simulink model "mit_ctl_Harness1"  (R2023a)
settings: configuration reference "config" (kept outside this file)
settings Model: DataDictionary=model_config.sldd  Creator=Administrator  LastModifiedBy=Administrator
settings ConfigSetRef: SourceName=config

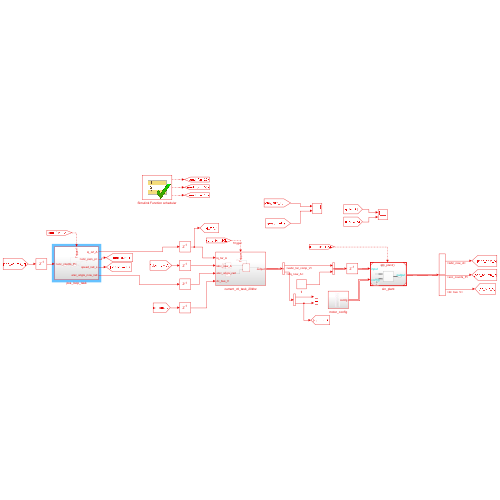
[thumbnail: Simulink's stored preview of the top-level diagram]
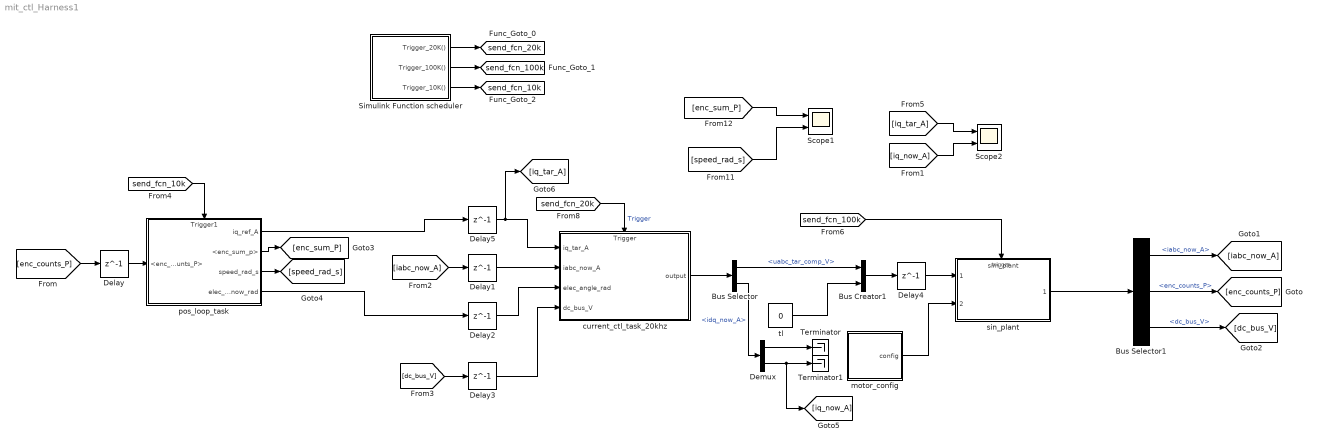
== system mit_ctl_Harness1 ==
  Bus Creator1 : BusCreator  Inputs=2  OutDataTypeStr=Bus: SimPlantInput  NonVirtualBus=on
      settings: InheritFromInputs=off
  Bus Selector : BusSelector  OutputSignals=uabc_tar_comp_V,idq_now_A
  Bus Selector1 : BusSelector  OutputSignals=iabc_now_A,enc_counts_P,dc_bus_V
  Delay{,1..5} (6 alike) : Delay  DelayLength=1
  Demux : Demux  Outputs=2
  Scope1 : Scope  NumInputPorts=2
  Scope2 : Scope  NumInputPorts=2
  Simulink Function scheduler : Test Sequence  Tag=__SLT_FCN_CALL__  TreatAsAtomicUnit=on
  Terminator : Terminator
  Terminator1 : Terminator
  current_ctl_task_20khz : Subsystem
      settings: PortSchema="{\"entries\":[{\"content\":{\"sides\":[{\"content\":{\"connectorIds\":[\"In1\",\"In2\",\"In3\",\"In4\"]},\"type\":\"ConnectorPlacement.EquallySpacedRectSide\",\"uuid\":\"a5b1ef4d-2ad4-4f45-b086-2b039a0eea6e\"},{\"content\":{\"connectorIds\":[\"Out1\"],\"side\":\"RIGHT\"},\"type\":\"ConnectorPlacement.EquallySpacedRectSide\",\"uuid\":\"557b3bf9-18ae-4636-b21a-b42dc238cf2f\"},{\"content\":{\"connectorIds\":[\"In5\"],\"side\":\"TOP\"},\"type\":\"ConnectorPlacement.EquallySpacedRectSide\",\"uuid\":\"c7c54502-1896-4674-886e-e49012a97e9f\"}]},\"type\":\"ConnectorPlacement.EquallySpacedConnector\",\"uuid\":\"12b1717b-20ca-4637-a661-7f52493678ac\"}],\"packageUris\":[\"http://schema.mathworks.com/mf0/Connector/R2020b\"],\"version\":\"1.0\"}"
  motor_config : Subsystem
  pos_loop_task : Subsystem
      settings: PortSchema="{\"entries\":[{\"content\":{\"sides\":[{\"content\":{\"connectorIds\":[\"In1\"]},\"type\":\"ConnectorPlacement.EquallySpacedRectSide\",\"uuid\":\"d22d2e99-a610-46a0-ab0a-73cacfeb4149\"},{\"content\":{\"connectorIds\":[\"Out1\",\"Out2\",\"Out3\",\"Out4\"],\"side\":\"RIGHT\"},\"type\":\"ConnectorPlacement.EquallySpacedRectSide\",\"uuid\":\"f98e4468-eff7-4a22-be49-e79447519cdd\"},{\"content\":{\"connectorIds\":[\"In2\"],\"side\":\"TOP\"},\"type\":\"ConnectorPlacement.EquallySpacedRectSide\",\"uuid\":\"8b4d848a-2398-4b91-b8fd-5654866e7819\"}]},\"type\":\"ConnectorPlacement.EquallySpacedConnector\",\"uuid\":\"8f3a11ef-b544-4005-a32a-da156990f746\"}],\"packageUris\":[\"http://schema.mathworks.com/mf0/Connector/R2020b\"],\"version\":\"1.0\"}"
  sin_plant : ModelReference  ModelNameDialog=sim_plant  SimulationMode=Normal  ModelReferenceVersion=1.108  TriggerPortName=Trigger  TriggerPortTriggerType=function-call  TriggerPortStatesWhenEnabling=held
  tl : Constant  Value=0  OutDataTypeStr=single  SampleTime=-1
  tag scope: send_fcn_100k=global, send_fcn_10k=global, send_fcn_20k=global
  wires:
  Simulink Function scheduler/1(Trigger_20K()) -> [send_fcn_20k]
  Simulink Function scheduler/2(Trigger_100K()) -> [send_fcn_100k]
  [send_fcn_100k] -> sin_plant/Trigger
  motor_config/1(config) -> sin_plant/2
  Bus Selector/1 -> Bus Creator1/1  "<uabc_tar_comp_V>"
  tl/1 -> Bus Creator1/2
  Bus Selector1/1 -> [iabc_now_A]  "<iabc_now_A>"
  Bus Selector1/3 -> [dc_bus_V]  "<dc_bus_V>"
  Simulink Function scheduler/3(Trigger_10K()) -> [send_fcn_10k]
  [send_fcn_20k] -> current_ctl_task_20khz/5(Trigger)  "Trigger"
  current_ctl_task_20khz/1(output) -> Bus Selector/1
  Bus Selector1/2 -> [enc_counts_P]  "<enc_counts_P>"
  Bus Selector/2 -> Demux/1  "<idq_now_A>"
  Demux/1 -> Terminator/1
  Demux/2 -> [iq_now_A], Terminator1/1
  [send_fcn_10k] -> pos_loop_task/2(Trigger1)
  pos_loop_task/2(<enc_sum_p>) -> [enc_sum_P]
  pos_loop_task/3(speed_rad_s) -> [speed_rad_s]
  [enc_counts_P] -> Delay/1
  [iabc_now_A] -> Delay1/1
  pos_loop_task/4(elec_angle_now_rad) -> Delay2/1
  Bus Creator1/1 -> Delay4/1
  pos_loop_task/1(iq_ref_A) -> Delay5/1
  Delay1/1 -> current_ctl_task_20khz/2(iabc_now_A)
  Delay2/1 -> current_ctl_task_20khz/3(elec_angle_rad)
  [dc_bus_V] -> Delay3/1
  sin_plant/1 -> Bus Selector1/1
  Delay/1 -> pos_loop_task/1(<enc_counts_P>)
  [enc_sum_P] -> Scope1/1
  [speed_rad_s] -> Scope1/2
  Delay3/1 -> current_ctl_task_20khz/4(dc_bus_V)
  Delay4/1 -> sin_plant/1
  [iq_tar_A] -> Scope2/1
  [iq_now_A] -> Scope2/2
  Delay5/1 -> [iq_tar_A], current_ctl_task_20khz/1(iq_tar_A)

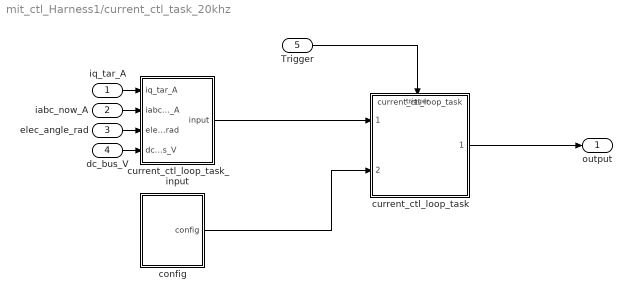
== system mit_ctl_Harness1/current_ctl_task_20khz ==
  iq_tar_A : Inport
  iabc_now_A : Inport  Port=2
  elec_angle_rad : Inport  Port=3
  dc_bus_V : Inport  Port=4
  Trigger : Inport  Port=5
  config : Subsystem
  current_ctl_loop_task : ModelReference  ModelNameDialog=current_ctl_loop_task  SimulationMode=Normal  ModelReferenceVersion=2.1046  TriggerPortName=Trigger  TriggerPortTriggerType=function-call  TriggerPortStatesWhenEnabling=held
  current_ctl_loop_task_input : Subsystem
  output : Outport
  wires:
  elec_angle_rad/1 -> current_ctl_loop_task_input/3(elec_angle_rad)
  dc_bus_V/1 -> current_ctl_loop_task_input/4(dc_bus_V)
  Trigger/1 -> current_ctl_loop_task/Trigger
  iq_tar_A/1 -> current_ctl_loop_task_input/1(iq_tar_A)
  iabc_now_A/1 -> current_ctl_loop_task_input/2(iabc_now_A)
  current_ctl_loop_task_input/1(input) -> current_ctl_loop_task/1
  config/1(config) -> current_ctl_loop_task/2
  current_ctl_loop_task/1 -> output/1

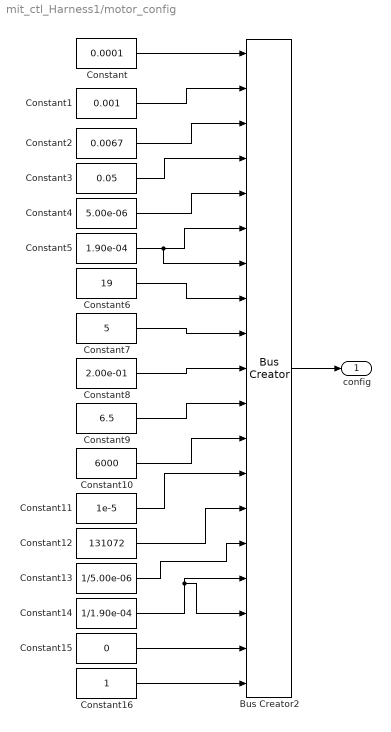
== system mit_ctl_Harness1/motor_config ==
  Bus Creator2 : BusCreator  Inputs=19  OutDataTypeStr=Bus: SimPlantConfig  NonVirtualBus=on
      settings: InheritFromInputs=off
  Constant : Constant  Value=0.0001  OutDataTypeStr=single
  Constant1 : Constant  Value=0.001  OutDataTypeStr=single
  Constant10 : Constant  Value=6000  OutDataTypeStr=single
  Constant11 : Constant  Value=1e-5  OutDataTypeStr=single
  Constant12 : Constant  Value=131072  OutDataTypeStr=uint32
  Constant13 : Constant  Value=1/5.00e-06  OutDataTypeStr=single
  Constant14 : Constant  Value=1/1.90e-04  OutDataTypeStr=single
  Constant15 : Constant  Value=0  OutDataTypeStr=int64
  Constant16 : Constant  OutDataTypeStr=single
  Constant2 : Constant  Value=0.0067  OutDataTypeStr=single
  Constant3 : Constant  Value=0.05  OutDataTypeStr=single
  Constant4 : Constant  Value=5.00e-06  OutDataTypeStr=single
  Constant5 : Constant  Value=1.90e-04  OutDataTypeStr=single
  Constant6 : Constant  Value=19  OutDataTypeStr=single
  Constant7 : Constant  Value=5  OutDataTypeStr=single
  Constant8 : Constant  Value=2.00e-01  OutDataTypeStr=single
  Constant9 : Constant  Value=6.5  OutDataTypeStr=single
  config : Outport
  wires:
  Bus Creator2/1 -> config/1
  Constant/1 -> Bus Creator2/1
  Constant1/1 -> Bus Creator2/2
  Constant2/1 -> Bus Creator2/3
  Constant3/1 -> Bus Creator2/4
  Constant4/1 -> Bus Creator2/5
  Constant5/1 -> Bus Creator2/6, Bus Creator2/7
  Constant6/1 -> Bus Creator2/8
  Constant7/1 -> Bus Creator2/9
  Constant8/1 -> Bus Creator2/10
  Constant9/1 -> Bus Creator2/11
  Constant10/1 -> Bus Creator2/12
  Constant11/1 -> Bus Creator2/13
  Constant12/1 -> Bus Creator2/14
  Constant13/1 -> Bus Creator2/15
  Constant14/1 -> Bus Creator2/17, Bus Creator2/16
  Constant15/1 -> Bus Creator2/18
  Constant16/1 -> Bus Creator2/19

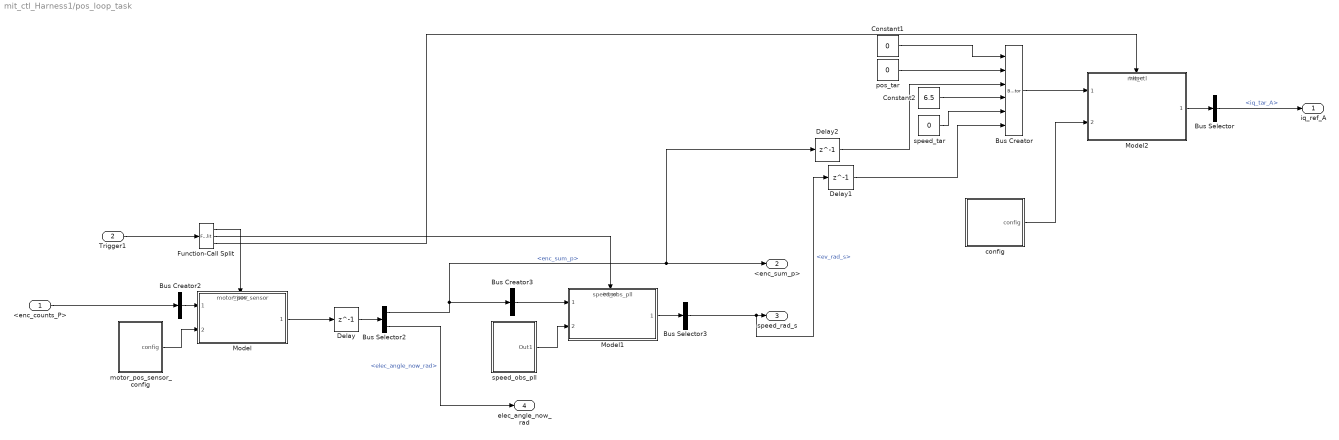
== system mit_ctl_Harness1/pos_loop_task ==
  <enc_counts_P> : Inport
  Trigger1 : Inport  Port=2
  Bus Creator : BusCreator  Inputs=6  OutDataTypeStr=Bus: MitCtlInput  NonVirtualBus=on
      settings: InheritFromInputs=off
  Bus Creator2 : BusCreator  Inputs=1  OutDataTypeStr=Bus: MotorPosSensorInput  NonVirtualBus=on
      settings: InheritFromInputs=off
  Bus Creator3 : BusCreator  Inputs=1  OutDataTypeStr=Bus: SpeedObsPllInput  NonVirtualBus=on
      settings: InheritFromInputs=off
  Bus Selector : BusSelector  OutputSignals=iq_tar_A
  Bus Selector2 : BusSelector  OutputSignals=enc_sum_p,elec_angle_now_rad
  Bus Selector3 : BusSelector  OutputSignals=ev_rad_s
  Constant1 : Constant  Value=0  OutDataTypeStr=single
  Constant2 : Constant  Value=6.5  OutDataTypeStr=single
  Delay : Delay  DelayLength=1
  Delay1 : Delay  DelayLength=1
  Delay2 : Delay  DelayLength=1
  Function-Call Split : FunctionCallSplit  IconShape=distinctive  NumOutputPorts=3  OutputPortLayout=default
  Model : ModelReference  ModelNameDialog=motor_pos_sensor  SimulationMode=Normal  ModelReferenceVersion=2.961  TriggerPortName=Trigger  TriggerPortTriggerType=function-call  TriggerPortStatesWhenEnabling=held
  Model1 : ModelReference  ModelNameDialog=speed_obs_pll  UsingDefaultArgumentValue=0,0,0  SimulationMode=Normal  ModelReferenceVersion=2.279  TriggerPortName=Trigger  TriggerPortTriggerType=function-call  TriggerPortStatesWhenEnabling=held
  Model2 : ModelReference  ModelNameDialog=mit_ctl.slx  SimulationMode=Normal  ModelReferenceVersion=2.992  TriggerPortName=Trigger  TriggerPortTriggerType=function-call  TriggerPortStatesWhenEnabling=held
  config : Subsystem
  motor_pos_sensor_config : Subsystem
  pos_tar : Constant  Value=0  OutDataTypeStr=int64
  speed_obs_pll : Subsystem
  speed_tar : Constant  Value=0  OutDataTypeStr=single
  iq_ref_A : Outport
  <enc_sum_p> : Outport  Port=2
  speed_rad_s : Outport  Port=3
  elec_angle_now_rad : Outport  Port=4
  wires:
  Bus Selector3/1 -> Delay1/1, speed_rad_s/1  "<ev_rad_s>"
  Model1/1 -> Bus Selector3/1
  motor_pos_sensor_config/1(config) -> Model/2
  speed_obs_pll/1(Out1) -> Model1/2
  Bus Selector2/1 -> Bus Creator3/1, Delay2/1, <enc_sum_p>/1  "<enc_sum_p>"
  Bus Creator2/1 -> Model/1
  Bus Selector2/2 -> elec_angle_now_rad/1  "<elec_angle_now_rad>"
  Trigger1/1 -> Function-Call Split/1
  Function-Call Split/1 -> Model/Trigger
  Function-Call Split/2 -> Model1/Trigger
  Bus Creator3/1 -> Model1/1
  <enc_counts_P>/1 -> Bus Creator2/1
  Model/1 -> Delay/1
  Delay/1 -> Bus Selector2/1
  Function-Call Split/3 -> Model2/Trigger
  pos_tar/1 -> Bus Creator/2
  Constant1/1 -> Bus Creator/1
  Bus Selector/1 -> iq_ref_A/1  "<iq_tar_A>"
  Delay1/1 -> Bus Creator/6
  Delay2/1 -> Bus Creator/3
  Model2/1 -> Bus Selector/1
  config/1(config) -> Model2/2
  Bus Creator/1 -> Model2/1
  speed_tar/1 -> Bus Creator/5
  Constant2/1 -> Bus Creator/4

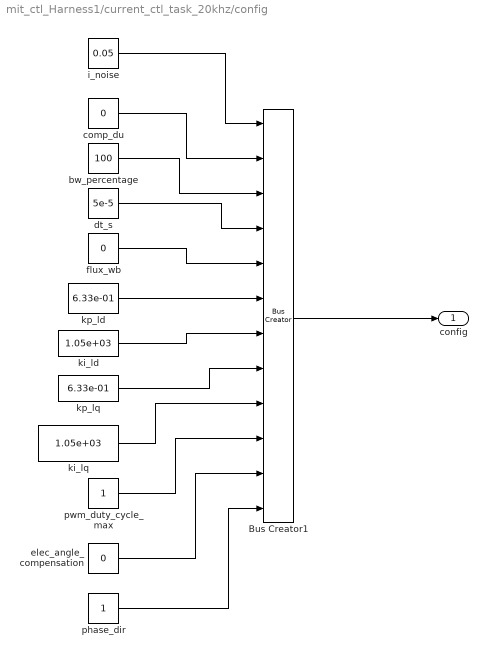
== system mit_ctl_Harness1/current_ctl_task_20khz/config ==
  Bus Creator1 : BusCreator  Inputs=12  OutDataTypeStr=Bus: CurrentCtlConfig  NonVirtualBus=on
      settings: InheritFromInputs=off
  bw_percentage : Constant  Value=100  OutDataTypeStr=single
  comp_du : Constant  Value=0  OutDataTypeStr=single
  dt_s : Constant  Value=5e-5  OutDataTypeStr=single
  elec_angle_compensation : Constant  Value=0  OutDataTypeStr=single
  flux_wb : Constant  Value=0  OutDataTypeStr=single
  i_noise : Constant  Value=0.05  OutDataTypeStr=single
  ki_ld : Constant  Value=1.05e+03  OutDataTypeStr=single
  ki_lq : Constant  Value=1.05e+03  OutDataTypeStr=single
  kp_ld : Constant  Value=6.33e-01  OutDataTypeStr=single
  kp_lq : Constant  Value=6.33e-01  OutDataTypeStr=single
  phase_dir : Constant  OutDataTypeStr=int8  LockScale=on
  pwm_duty_cycle_max : Constant  OutDataTypeStr=single
  config : Outport
  wires:
  flux_wb/1 -> Bus Creator1/5
  pwm_duty_cycle_max/1 -> Bus Creator1/10
  comp_du/1 -> Bus Creator1/2
  bw_percentage/1 -> Bus Creator1/3
  elec_angle_compensation/1 -> Bus Creator1/11
  i_noise/1 -> Bus Creator1/1
  Bus Creator1/1 -> config/1
  kp_lq/1 -> Bus Creator1/8
  ki_ld/1 -> Bus Creator1/7
  phase_dir/1 -> Bus Creator1/12
  kp_ld/1 -> Bus Creator1/6
  ki_lq/1 -> Bus Creator1/9
  dt_s/1 -> Bus Creator1/4

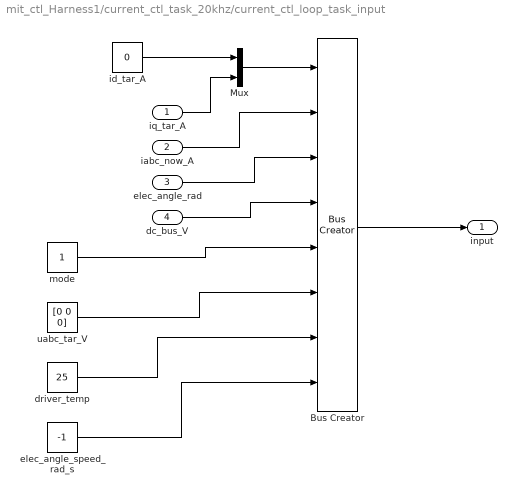
== system mit_ctl_Harness1/current_ctl_task_20khz/current_ctl_loop_task_input ==
  iq_tar_A : Inport
  iabc_now_A : Inport  Port=2
  elec_angle_rad : Inport  Port=3
  dc_bus_V : Inport  Port=4
  Bus Creator : BusCreator  Inputs=8  OutDataTypeStr=Bus: CurrentCtlInput  NonVirtualBus=on
      settings: InheritFromInputs=off
  Mux : Mux  Inputs=2
  driver_temp : Constant  Value=25  OutDataTypeStr=single  SampleTime=-1
  elec_angle_speed_rad_s : Constant  Value=-1  OutDataTypeStr=single  SampleTime=-1
  id_tar_A : Constant  Value=0  OutDataTypeStr=single  SampleTime=-1
  mode : Constant  OutDataTypeStr=uint8  SampleTime=-1
  uabc_tar_V : Constant  Value=[0 0 0]  OutDataTypeStr=single  SampleTime=-1
  input : Outport
  wires:
  Mux/1 -> Bus Creator/1
  Bus Creator/1 -> input/1
  dc_bus_V/1 -> Bus Creator/4
  iabc_now_A/1 -> Bus Creator/2
  elec_angle_rad/1 -> Bus Creator/3
  iq_tar_A/1 -> Mux/2
  id_tar_A/1 -> Mux/1
  mode/1 -> Bus Creator/5
  uabc_tar_V/1 -> Bus Creator/6
  driver_temp/1 -> Bus Creator/7
  elec_angle_speed_rad_s/1 -> Bus Creator/8

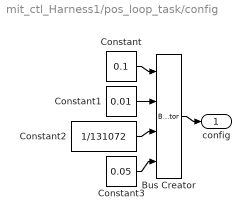
== system mit_ctl_Harness1/pos_loop_task/config ==
  Bus Creator : BusCreator  Inputs=4  OutDataTypeStr=Bus: MitCtlConfig  NonVirtualBus=on
      settings: InheritFromInputs=off
  Constant : Constant  Value=0.1  OutDataTypeStr=single
  Constant1 : Constant  Value=0.01  OutDataTypeStr=single
  Constant2 : Constant  Value=1/131072  OutDataTypeStr=single
  Constant3 : Constant  Value=0.05  OutDataTypeStr=single
  config : Outport
  wires:
  Bus Creator/1 -> config/1
  Constant1/1 -> Bus Creator/2
  Constant/1 -> Bus Creator/1
  Constant2/1 -> Bus Creator/3
  Constant3/1 -> Bus Creator/4

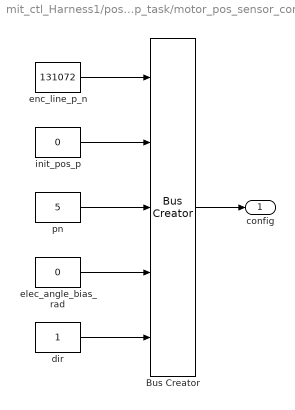
== system mit_ctl_Harness1/pos_loop_task/motor_pos_sensor_config ==
  Bus Creator : BusCreator  Inputs=5  OutDataTypeStr=Bus: MotorPosSensorConfig  NonVirtualBus=on
      settings: InheritFromInputs=off
  dir : Constant  OutDataTypeStr=int8
  elec_angle_bias_rad : Constant  Value=0  OutDataTypeStr=single
  enc_line_p_n : Constant  Value=131072  OutDataTypeStr=uint32
  init_pos_p : Constant  Value=0  OutDataTypeStr=int64
  pn : Constant  Value=5  OutDataTypeStr=uint32
  config : Outport
  wires:
  Bus Creator/1 -> config/1
  enc_line_p_n/1 -> Bus Creator/1
  pn/1 -> Bus Creator/3
  init_pos_p/1 -> Bus Creator/2
  elec_angle_bias_rad/1 -> Bus Creator/4
  dir/1 -> Bus Creator/5

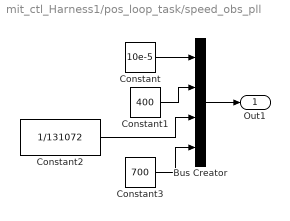
== system mit_ctl_Harness1/pos_loop_task/speed_obs_pll ==
  Bus Creator : BusCreator  Inputs=4  OutDataTypeStr=Bus: SpeedObsPllConfig  NonVirtualBus=on
      settings: InheritFromInputs=off
  Constant : Constant  Value=10e-5  OutDataTypeStr=single
  Constant1 : Constant  Value=400  OutDataTypeStr=single
  Constant2 : Constant  Value=1/131072  OutDataTypeStr=single
  Constant3 : Constant  Value=700  OutDataTypeStr=single
  Out1 : Outport
  wires:
  Bus Creator/1 -> Out1/1
  Constant/1 -> Bus Creator/1
  Constant1/1 -> Bus Creator/2
  Constant2/1 -> Bus Creator/3
  Constant3/1 -> Bus Creator/4

== stateflow chart mit_ctl_Harness1/Simulink Function scheduler ==
  settings: updateMethod=DISCRETE  sampleTime=1.0E-5
  state Run
    num = 0;
    pos_num = 0;
    send(Trigger_10K);
    send(Trigger_20K);
    send(Trigger_100K);
  state step_1
    num = num +1;
    pos_num = pos_num+1;
    if (num >= 5)
    send(Trigger_20K);
    num  = 0;
    end
    if (pos_num>= 10)
    send(Trigger_10K);
    pos_num= 0;
    end
    send(Trigger_100K);
    settings: description="产生100k  20k  10k 函数周期调用"
  (default) -> Run
  Run -> step_1 : [
      | true
      | ]
  step_1 -> Run : [
      | false
      | ]
  data: num local; pos_num local
  events: Trigger_20K output FUNCTION_CALL_EVENT; Trigger_100K output FUNCTION_CALL_EVENT; Trigger_10K output FUNCTION_CALL_EVENT
